simulink model "NLT"  (R2021a)
settings: Solver=VariableStepAuto  StartTime=0.0  StopTime=10.0  RelTol=1e-3
settings Model: Creator=Sirius  LastModifiedBy=Sirius

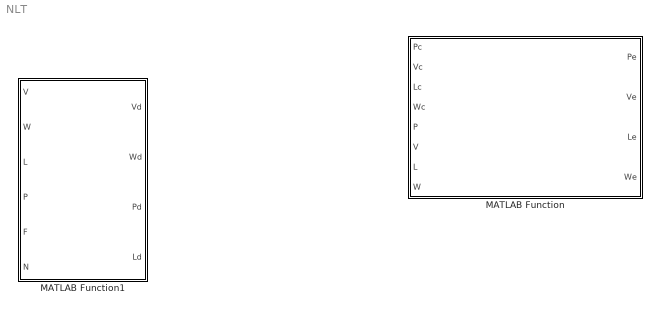
== system NLT ==
  MATLAB Function : MATLAB Function  TreatAsAtomicUnit=on
  MATLAB Function1 : MATLAB Function  TreatAsAtomicUnit=on

== matlab function NLT/MATLAB Function1 ==
  data: V input; Vd output; W input; L input; P input; F input; N input; Wd output; Pd output; Ld output
function [Vd,Wd,Pd,Ld] = QRotor(V,W,L,P,F,N)
Vd=-Skew(W)*V+1/m*F;
Wd=Jinv*Skew(W)*J*W+Jinv*N;
Pd=RPY2Rmat(L)*V;
Ld=RPY2Qmat(L)*W;
end

== matlab function NLT/MATLAB Function ==
  data: Pc input; Pe output; Vc input; Lc input; Wc input; P input; V input; L input; W input; Ve output; Le output; We output
function [Pe,Ve,Le,We] = NLT(Pc,Vc,Lc,Wc,P,V,L,W)
R=RPY2Rmat(L);
Rt=R';
Rc=RPY2Rmat(Lc);


Ve=V-Vc;
We=W-Wc;
Pe=Rt*(P-Pc);
%Rc:C->I
%R:B->I
Le=Rmat2PRY(Rc'*R);
